simulink model "Model"  (R2023a)
settings: Solver=VariableStepAuto  StartTime=0.0  StopTime=10.0  RelTol=1e-3
values from neighbouring files (symbols this model uses):
  A = [0 1 0 0 0 0 ... (first row only)    [kf.m]
undefined symbols (not defined in the file or in its folder): B, x0
settings Model: Creator=mluser  LastModifiedBy=mluser

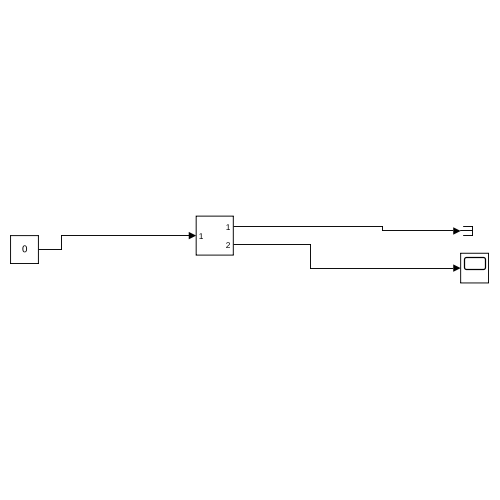
[thumbnail: Simulink's stored preview of the top-level diagram]
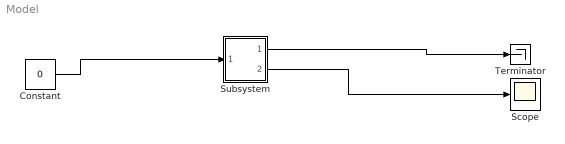
== system Model ==
  Constant : Constant  Value=0
  Scope : Scope
  Subsystem : Subsystem
  Terminator : Terminator
  wires:
  Constant/1 -> Subsystem/1(In1)
  Subsystem/1(Out1) -> Terminator/1
  Subsystem/2(Out2) -> Scope/1

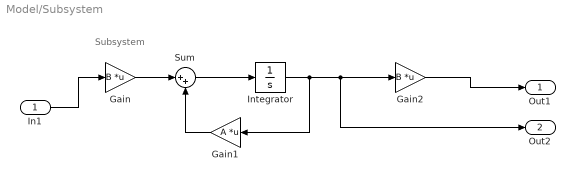
== system Model/Subsystem ==
  note: Subsystem
  In1 : Inport
  Gain : Gain  Gain=B  Multiplication=Matrix(K*u)
  Gain1 : Gain  Gain=A  Multiplication=Matrix(K*u)
  Gain2 : Gain  Gain=B  Multiplication=Matrix(K*u)
  Integrator : Integrator  InitialCondition=x0
  Sum : Sum  Inputs=|++
  Out1 : Outport
  Out2 : Outport  Port=2
  wires:
  Gain1/1 -> Sum/2
  Gain/1 -> Sum/1
  In1/1 -> Gain/1
  Integrator/1 -> Out2/1, Gain2/1, Gain1/1
  Sum/1 -> Integrator/1
  Gain2/1 -> Out1/1
